simulink model "SecRwRtStFwdBkwdIsPosChk"  (R2024b)
settings: Solver=FixedStepDiscrete  StartTime=0.0  StopTime=10.0  FixedStep=0.01  RelTol=1e-3
undefined symbols (not defined in the file or in its folder): KeSMSuSecRwStFwdBkwdPosDelta_Val, KeSMSuSecRwStFwdBkwdPosTolr_Val
libraries: StIsPosChkLib x16, simulink x8
(part 1 of 2)
settings Model: Creator=sn2xws  LastModifiedBy=sn55gm
settings Model: ModifiedHistory=|
  | 2023.8.1 V2.0.0 CR421790 增加模式21-26
  | 2023.9.14 V2.1.0 Bug 540886 修改亲密模式判断到位的条件为10ms周期计算
  | 2023.11.16  V2.3.0 Issue 566045 全躺，vip，腿托打开增加前后位置
  | 2024.7.9 V3.0.0 557模式流程V1.9
  | 2024.8.15 V3.0.1 智享模式需要计算目标位置，不能直接判断到位置，posalready赋值0
  | 2024.9.5 V3.0.2 新增Md56，注释不用的模式
  | 2024.9.13 V3.0.3 6s版本lug不动二排前后
  | 2024.10.14 V3.0.4 新增Md57，md58
  | 2024.11.27 V3.0.5 Md57运行时，不能直接判断到位置
  | 25.7.1 V3.13.0 新增Md61 Md62
settings SolverCC: AlgebraicLoopSolver=TrustRegion
settings DataIOCC: SaveFormat=StructureWithTime  ReturnWorkspaceOutputs=off
settings OptimizationCC: DefaultParameterBehavior=Inlined  EnhancedBackFolding=on  PassReuseOutputArgsAs=Individual arguments  ZeroExternalMemoryAtStartup=off  ZeroInternalMemoryAtStartup=off  OptimizeBlockOrder=speed  DifferentSizesBufferReuse=on  OptimizationCustomize=off  EfficientTunableParamExpr=on
settings DebuggingCC: ParameterTunabilityLossMsg=error  UnconnectedInputMsg=warning  UnconnectedOutputMsg=warning  UnconnectedLineMsg=warning  ArithmeticOperatorsInVariantConditions=warning
settings ModelReferenceCC: EnableRefExpFcnMdlSchedulingChecks=on  ModelReferenceNumInstancesAllowed=Single
settings SFSimCC: MATLABDynamicMemAlloc=off  CustomCodeUndefinedFunction=UseInterfaceOnly
settings RTWCC: Description=AUTOSAR  SystemTargetFile=autosar.tlc  GenCodeOnly=on  TemplateMakefile=ert_default_tmf  GenerateReport=on  IncludeHyperlinkInReport=on  LaunchReport=on  DataTypeReplacement=CDataTypesFixedWidth  GenerateTraceInfo=on  GenerateTraceReport=on  GenerateTraceReportSl=on  GenerateTraceReportSf=on  GenerateTraceReportEml=on  GPUComputeCapability=3.5
settings CodeAppCC: ForceParamTrailComments=on  IgnoreCustomStorageClasses=off  OperatorAnnotations=on  SimulinkDataObjDesc=on  SFDataObjDesc=on  InsertBlockDesc=on
settings STFCustomTargetCC: TargetLangStandard=C99 (ISO)  MultiwordLength=256  ParMdlRefBuildCompliant=on  CompOptLevelCompliant=on  IncludeMdlTerminateFcn=off  CombineOutputUpdateFcns=on  SuppressErrorStatus=on  ERTCustomFileBanners=on  SupportNonFinite=off  SupportComplex=off  SupportContinuousTime=off  SupportNonInlinedSFcns=off  RemoveResetFunc=on  MATLABClassNameForMDSCustomization=Simulink.SoftwareTarget.ERTCustomization  AutosarCompliant=on  UseToolchainInfoCompliant=on  LookupTableObjectStructAxisOrder=2,1,3,4,...  LUTObjectStructOrderEvenSpacing=Size,Table,Breakpoints  SystemTargetFile=autosar.tlc
settings ERTTargetCC: TargetLangStandard=C99 (ISO)  ConcurrentExecutionCompliant=off  IncludeMdlTerminateFcn=off  SuppressErrorStatus=on  SupportNonFinite=off  SupportComplex=off  ModelStepFunctionPrototypeControlCompliant=off  CPPClassGenCompliant=off  AutosarCompliant=on  LookupTableObjectStructAxisOrder=2,1,3,4,...  LUTObjectStructOrderEvenSpacing=Size,Table,Breakpoints  ERTCustomFileTemplate=example_file_process.tlc  ERTFilePackagingFormat=Compact  BooleanTrueId=TRUE  BooleanFalseId=FALSE  DynamicArrayContainerType=coder::array

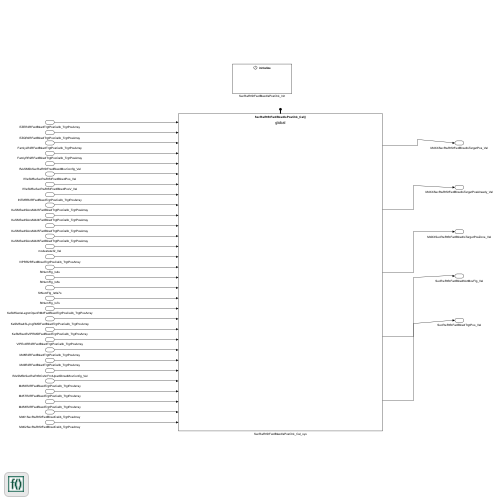
[thumbnail: Simulink's stored preview of the top-level diagram]
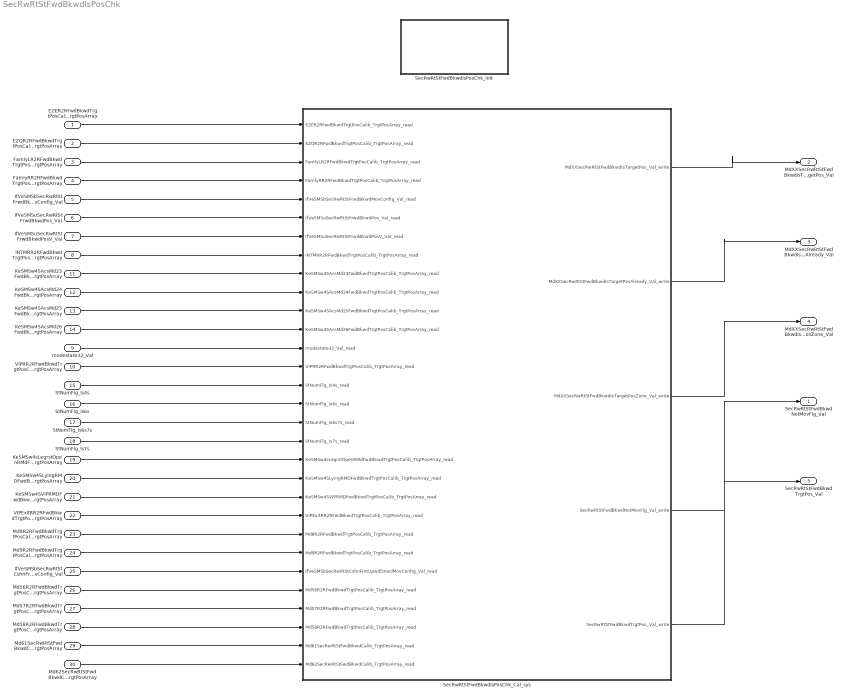
== system SecRwRtStFwdBkwdIsPosChk ==
  EZER2RFwdBkwdTrgtPosCalib_TrgtPosArray : Inport  Description=|  OutDataTypeStr=uint16  PortDimensions=3
      | 0:Pos
      | 1:Max
      | 2:Min
  EZQR2RFwdBkwdTrgtPosCalib_TrgtPosArray : Inport  Description=|  Port=2  OutDataTypeStr=uint16  PortDimensions=3
      | 0:Pos
      | 1:Max
      | 2:Min
  FamlyLR2RFwdBkwdTrgtPosCalib_TrgtPosArray : Inport  Description=|  Port=3  OutDataTypeStr=uint16  PortDimensions=3
      | 0:Pos
      | 1:Max
      | 2:Min
  FamlyRR2RFwdBkwdTrgtPosCalib_TrgtPosArray : Inport  Description=|  Port=4  OutDataTypeStr=uint16  PortDimensions=3
      | 0:Pos
      | 1:Max
      | 2:Min
  IfVeSMSbSecRwRtStFrwdBkwdMovConfig_Val : Inport  Port=5  OutDataTypeStr=boolean  PortDimensions=1
  IfVeSMSuSecRwRtStFrwdBkwdPos_Val : Inport  Port=6  OutDataTypeStr=uint16  PortDimensions=1
  IfVeSMSuSecRwRtStFrwdBkwdPosV_Val : Inport  Port=7  OutDataTypeStr=boolean  PortDimensions=1
  INTMRR2RFwdBkwdTrgtPosCalib_TrgtPosArray : Inport  Description=|  Port=8  OutDataTypeStr=uint16  PortDimensions=3
      | 0:Pos
      | 1:Max
      | 2:Min
  modestate32_Val : Inport  Port=9  OutDataTypeStr=uint32  PortDimensions=1
  VIPRR2RFwdBkwdTrgtPosCalib_TrgtPosArray : Inport  Description=|  Port=10  OutDataTypeStr=uint16  PortDimensions=3
      | 0:Pos
      | 1:Max
      | 2:Min
  KeSMSw4SAcsMd23FwdBkwdTrgtPosCalib_TrgtPosArray : Inport  Description=|  Port=11  OutDataTypeStr=uint16  PortDimensions=3
      | 0:Pos
      | 1:Max
      | 2:Min
  KeSMSw4SAcsMd24FwdBkwdTrgtPosCalib_TrgtPosArray : Inport  Description=|  Port=12  OutDataTypeStr=uint16  PortDimensions=3
      | 0:Pos
      | 1:Max
      | 2:Min
  KeSMSw4SAcsMd25FwdBkwdTrgtPosCalib_TrgtPosArray : Inport  Description=|  Port=13  OutDataTypeStr=uint16  PortDimensions=3
      | 0:Pos
      | 1:Max
      | 2:Min
  KeSMSw4SAcsMd26FwdBkwdTrgtPosCalib_TrgtPosArray : Inport  Description=|  Port=14  OutDataTypeStr=uint16  PortDimensions=3
      | 0:Pos
      | 1:Max
      | 2:Min
  StNumFlg_Is4s : Inport  Port=15  OutDataTypeStr=boolean  PortDimensions=1
  StNumFlg_Is6s : Inport  Port=16  OutDataTypeStr=boolean  PortDimensions=1
  StNumFlg_Is6s7s : Inport  Port=17  OutDataTypeStr=boolean  PortDimensions=1
  StNumFlg_Is7s : Inport  Port=18  OutDataTypeStr=boolean  PortDimensions=1
  KeSMSw4sLegrstOpenRMdFwdBkwdTrgtPosCalib_TrgtPosArray : Inport  Description=|  Port=19  OutDataTypeStr=uint16  PortDimensions=3
      | 0:Pos
      | 1:Max
      | 2:Min
  KeSMSw4SLyingRMDFwdBkwdTrgtPosCalib_TrgtPosArray : Inport  Description=|  Port=20  OutDataTypeStr=uint16  PortDimensions=3
      | 0:Pos
      | 1:Max
      | 2:Min
  KeSMSw4SVIPRMDFwdBkwdTrgtPosCalib_TrgtPosArray : Inport  Description=|  Port=21  OutDataTypeStr=uint16  PortDimensions=3
      | 0:Pos
      | 1:Max
      | 2:Min
  VIPExitRR2RFwdBkwdTrgtPosCalib_TrgtPosArray : Inport  Description=|  Port=22  OutDataTypeStr=uint16  PortDimensions=3
      | 0:Pos
      | 1:Max
      | 2:Min
  Md8R2RFwdBkwdTrgtPosCalib_TrgtPosArray : Inport  Description=|  Port=23  OutDataTypeStr=uint16  PortDimensions=3
      | 0:Pos
      | 1:Max
      | 2:Min
  Md9R2RFwdBkwdTrgtPosCalib_TrgtPosArray : Inport  Description=|  Port=24  OutDataTypeStr=uint16  PortDimensions=3
      | 0:Pos
      | 1:Max
      | 2:Min
  IfVeSMSbSecRwRtStCshnFrntUpwdDnwdMovConfig_Val : Inport  Port=25  OutDataTypeStr=boolean  PortDimensions=1
  Md56R2RFwdBkwdTrgtPosCalib_TrgtPosArray : Inport  Description=|  Port=26  OutDataTypeStr=uint16  PortDimensions=3
      | 0:Pos
      | 1:Max
      | 2:Min
  Md57R2RFwdBkwdTrgtPosCalib_TrgtPosArray : Inport  Description=|  Port=27  OutDataTypeStr=uint16  PortDimensions=3
      | 0:Pos
      | 1:Max
      | 2:Min
  Md58R2RFwdBkwdTrgtPosCalib_TrgtPosArray : Inport  Description=|  Port=28  OutDataTypeStr=uint16  PortDimensions=3
      | 0:Pos
      | 1:Max
      | 2:Min
  Md61SecRwRtStFwdBkwdCalib_TrgtPosArray : Inport  Description=|  Port=29  OutDataTypeStr=uint16  PortDimensions=3
      | 0:Pos
      | 1:Max
      | 2:Min
  Md62SecRwRtStFwdBkwdCalib_TrgtPosArray : Inport  Description=|  Port=30  OutDataTypeStr=uint16  PortDimensions=3
      | 0:Pos
      | 1:Max
      | 2:Min
  SecRwRtStFwdBkwdIsPosChk_Cal_sys : Subsystem
  SecRwRtStFwdBkwdIsPosChk_Init : Subsystem
  SecRwRtStFwdBkwdNotMovFlg_Val : Outport  OutDataTypeStr=boolean  PortDimensions=1  VectorParamsAs1DForOutWhenUnconnected=off
  MdXXSecRwRtStFwdBkwdIsTargetPos_Val : Outport  Port=2  OutDataTypeStr=uint32  PortDimensions=1  VectorParamsAs1DForOutWhenUnconnected=off
  MdXXSecRwRtStFwdBkwdIsTargetPosAlready_Val : Outport  Port=3  OutDataTypeStr=uint32  PortDimensions=1  VectorParamsAs1DForOutWhenUnconnected=off
  MdXXSecRwRtStFwdBkwdIsTargetPosZone_Val : Outport  Port=4  OutDataTypeStr=uint32  PortDimensions=1  VectorParamsAs1DForOutWhenUnconnected=off
  SecRwRtStFwdBkwdTrgtPos_Val : Outport  Port=5  OutDataTypeStr=uint16  PortDimensions=1  VectorParamsAs1DForOutWhenUnconnected=off
  wires:
  EZER2RFwdBkwdTrgtPosCalib_TrgtPosArray/1 -> SecRwRtStFwdBkwdIsPosChk_Cal_sys/1(EZER2RFwdBkwdTrgtPosCalib_TrgtPosArray_read)
  EZQR2RFwdBkwdTrgtPosCalib_TrgtPosArray/1 -> SecRwRtStFwdBkwdIsPosChk_Cal_sys/2(EZQR2RFwdBkwdTrgtPosCalib_TrgtPosArray_read)
  FamlyLR2RFwdBkwdTrgtPosCalib_TrgtPosArray/1 -> SecRwRtStFwdBkwdIsPosChk_Cal_sys/3(FamlyLR2RFwdBkwdTrgtPosCalib_TrgtPosArray_read)
  FamlyRR2RFwdBkwdTrgtPosCalib_TrgtPosArray/1 -> SecRwRtStFwdBkwdIsPosChk_Cal_sys/4(FamlyRR2RFwdBkwdTrgtPosCalib_TrgtPosArray_read)
  IfVeSMSbSecRwRtStFrwdBkwdMovConfig_Val/1 -> SecRwRtStFwdBkwdIsPosChk_Cal_sys/5(IfVeSMSbSecRwRtStFrwdBkwdMovConfig_Val_read)
  IfVeSMSuSecRwRtStFrwdBkwdPos_Val/1 -> SecRwRtStFwdBkwdIsPosChk_Cal_sys/6(IfVeSMSuSecRwRtStFrwdBkwdPos_Val_read)
  IfVeSMSuSecRwRtStFrwdBkwdPosV_Val/1 -> SecRwRtStFwdBkwdIsPosChk_Cal_sys/7(IfVeSMSuSecRwRtStFrwdBkwdPosV_Val_read)
  INTMRR2RFwdBkwdTrgtPosCalib_TrgtPosArray/1 -> SecRwRtStFwdBkwdIsPosChk_Cal_sys/8(INTMRR2RFwdBkwdTrgtPosCalib_TrgtPosArray_read)
  modestate32_Val/1 -> SecRwRtStFwdBkwdIsPosChk_Cal_sys/13(modestate32_Val_read)
  VIPRR2RFwdBkwdTrgtPosCalib_TrgtPosArray/1 -> SecRwRtStFwdBkwdIsPosChk_Cal_sys/14(VIPRR2RFwdBkwdTrgtPosCalib_TrgtPosArray_read)
  SecRwRtStFwdBkwdIsPosChk_Cal_sys/1(MdXXSecRwRtStFwdBkwdIsTargetPos_Val_write) -> MdXXSecRwRtStFwdBkwdIsTargetPos_Val/1
  SecRwRtStFwdBkwdIsPosChk_Cal_sys/2(MdXXSecRwRtStFwdBkwdIsTargetPosAlready_Val_write) -> MdXXSecRwRtStFwdBkwdIsTargetPosAlready_Val/1
  SecRwRtStFwdBkwdIsPosChk_Cal_sys/3(MdXXSecRwRtStFwdBkwdIsTargetPosZone_Val_write) -> MdXXSecRwRtStFwdBkwdIsTargetPosZone_Val/1
  SecRwRtStFwdBkwdIsPosChk_Cal_sys/4(SecRwRtStFwdBkwdNotMovFlg_Val_write) -> SecRwRtStFwdBkwdNotMovFlg_Val/1
  SecRwRtStFwdBkwdIsPosChk_Cal_sys/5(SecRwRtStFwdBkwdTrgtPos_Val_write) -> SecRwRtStFwdBkwdTrgtPos_Val/1
  KeSMSw4SAcsMd23FwdBkwdTrgtPosCalib_TrgtPosArray/1 -> SecRwRtStFwdBkwdIsPosChk_Cal_sys/9(KeSMSw4SAcsMd23FwdBkwdTrgtPosCalib_TrgtPosArray_read)
  KeSMSw4SAcsMd24FwdBkwdTrgtPosCalib_TrgtPosArray/1 -> SecRwRtStFwdBkwdIsPosChk_Cal_sys/10(KeSMSw4SAcsMd24FwdBkwdTrgtPosCalib_TrgtPosArray_read)
  KeSMSw4SAcsMd25FwdBkwdTrgtPosCalib_TrgtPosArray/1 -> SecRwRtStFwdBkwdIsPosChk_Cal_sys/11(KeSMSw4SAcsMd25FwdBkwdTrgtPosCalib_TrgtPosArray_read)
  KeSMSw4SAcsMd26FwdBkwdTrgtPosCalib_TrgtPosArray/1 -> SecRwRtStFwdBkwdIsPosChk_Cal_sys/12(KeSMSw4SAcsMd26FwdBkwdTrgtPosCalib_TrgtPosArray_read)
  StNumFlg_Is4s/1 -> SecRwRtStFwdBkwdIsPosChk_Cal_sys/15(StNumFlg_Is4s_read)
  StNumFlg_Is6s/1 -> SecRwRtStFwdBkwdIsPosChk_Cal_sys/16(StNumFlg_Is6s_read)
  StNumFlg_Is6s7s/1 -> SecRwRtStFwdBkwdIsPosChk_Cal_sys/17(StNumFlg_Is6s7s_read)
  StNumFlg_Is7s/1 -> SecRwRtStFwdBkwdIsPosChk_Cal_sys/18(StNumFlg_Is7s_read)
  KeSMSw4sLegrstOpenRMdFwdBkwdTrgtPosCalib_TrgtPosArray/1 -> SecRwRtStFwdBkwdIsPosChk_Cal_sys/19(KeSMSw4sLegrstOpenRMdFwdBkwdTrgtPosCalib_TrgtPosArray_read)
  KeSMSw4SLyingRMDFwdBkwdTrgtPosCalib_TrgtPosArray/1 -> SecRwRtStFwdBkwdIsPosChk_Cal_sys/20(KeSMSw4SLyingRMDFwdBkwdTrgtPosCalib_TrgtPosArray_read)
  KeSMSw4SVIPRMDFwdBkwdTrgtPosCalib_TrgtPosArray/1 -> SecRwRtStFwdBkwdIsPosChk_Cal_sys/21(KeSMSw4SVIPRMDFwdBkwdTrgtPosCalib_TrgtPosArray_read)
  VIPExitRR2RFwdBkwdTrgtPosCalib_TrgtPosArray/1 -> SecRwRtStFwdBkwdIsPosChk_Cal_sys/22(VIPExitRR2RFwdBkwdTrgtPosCalib_TrgtPosArray_read)
  Md8R2RFwdBkwdTrgtPosCalib_TrgtPosArray/1 -> SecRwRtStFwdBkwdIsPosChk_Cal_sys/23(Md8R2RFwdBkwdTrgtPosCalib_TrgtPosArray_read)
  Md9R2RFwdBkwdTrgtPosCalib_TrgtPosArray/1 -> SecRwRtStFwdBkwdIsPosChk_Cal_sys/24(Md9R2RFwdBkwdTrgtPosCalib_TrgtPosArray_read)
  IfVeSMSbSecRwRtStCshnFrntUpwdDnwdMovConfig_Val/1 -> SecRwRtStFwdBkwdIsPosChk_Cal_sys/25(IfVeSMSbSecRwRtStCshnFrntUpwdDnwdMovConfig_Val_read)
  Md56R2RFwdBkwdTrgtPosCalib_TrgtPosArray/1 -> SecRwRtStFwdBkwdIsPosChk_Cal_sys/26(Md56R2RFwdBkwdTrgtPosCalib_TrgtPosArray_read)
  Md57R2RFwdBkwdTrgtPosCalib_TrgtPosArray/1 -> SecRwRtStFwdBkwdIsPosChk_Cal_sys/27(Md57R2RFwdBkwdTrgtPosCalib_TrgtPosArray_read)
  Md58R2RFwdBkwdTrgtPosCalib_TrgtPosArray/1 -> SecRwRtStFwdBkwdIsPosChk_Cal_sys/28(Md58R2RFwdBkwdTrgtPosCalib_TrgtPosArray_read)
  Md61SecRwRtStFwdBkwdCalib_TrgtPosArray/1 -> SecRwRtStFwdBkwdIsPosChk_Cal_sys/29(Md61SecRwRtStFwdBkwdCalib_TrgtPosArray_read)
  Md62SecRwRtStFwdBkwdCalib_TrgtPosArray/1 -> SecRwRtStFwdBkwdIsPosChk_Cal_sys/30(Md62SecRwRtStFwdBkwdCalib_TrgtPosArray_read)

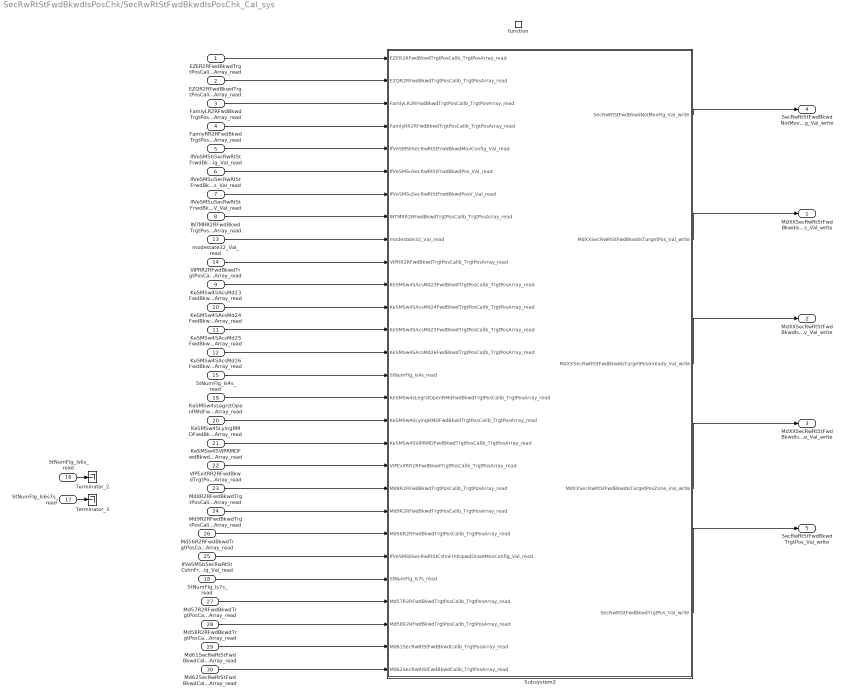
== system SecRwRtStFwdBkwdIsPosChk/SecRwRtStFwdBkwdIsPosChk_Cal_sys ==
  EZER2RFwdBkwdTrgtPosCalib_TrgtPosArray_read : Inport
  EZQR2RFwdBkwdTrgtPosCalib_TrgtPosArray_read : Inport  Port=2
  FamlyLR2RFwdBkwdTrgtPosCalib_TrgtPosArray_read : Inport  Port=3
  FamlyRR2RFwdBkwdTrgtPosCalib_TrgtPosArray_read : Inport  Port=4
  IfVeSMSbSecRwRtStFrwdBkwdMovConfig_Val_read : Inport  Port=5
  IfVeSMSuSecRwRtStFrwdBkwdPos_Val_read : Inport  Port=6
  IfVeSMSuSecRwRtStFrwdBkwdPosV_Val_read : Inport  Port=7
  INTMRR2RFwdBkwdTrgtPosCalib_TrgtPosArray_read : Inport  Port=8
  KeSMSw4SAcsMd23FwdBkwdTrgtPosCalib_TrgtPosArray_read : Inport  Port=9
  KeSMSw4SAcsMd24FwdBkwdTrgtPosCalib_TrgtPosArray_read : Inport  Port=10
  KeSMSw4SAcsMd25FwdBkwdTrgtPosCalib_TrgtPosArray_read : Inport  Port=11
  KeSMSw4SAcsMd26FwdBkwdTrgtPosCalib_TrgtPosArray_read : Inport  Port=12
  modestate32_Val_read : Inport  Port=13
  VIPRR2RFwdBkwdTrgtPosCalib_TrgtPosArray_read : Inport  Port=14
  StNumFlg_Is4s_read : Inport  Port=15
  StNumFlg_Is6s_read : Inport  Port=16
  StNumFlg_Is6s7s_read : Inport  Port=17
  StNumFlg_Is7s_read : Inport  Port=18
  KeSMSw4sLegrstOpenRMdFwdBkwdTrgtPosCalib_TrgtPosArray_read : Inport  Port=19
  KeSMSw4SLyingRMDFwdBkwdTrgtPosCalib_TrgtPosArray_read : Inport  Port=20
  KeSMSw4SVIPRMDFwdBkwdTrgtPosCalib_TrgtPosArray_read : Inport  Port=21
  VIPExitRR2RFwdBkwdTrgtPosCalib_TrgtPosArray_read : Inport  Port=22
  Md8R2RFwdBkwdTrgtPosCalib_TrgtPosArray_read : Inport  Port=23
  Md9R2RFwdBkwdTrgtPosCalib_TrgtPosArray_read : Inport  Port=24
  IfVeSMSbSecRwRtStCshnFrntUpwdDnwdMovConfig_Val_read : Inport  Port=25
  Md56R2RFwdBkwdTrgtPosCalib_TrgtPosArray_read : Inport  Port=26
  Md57R2RFwdBkwdTrgtPosCalib_TrgtPosArray_read : Inport  Port=27
  Md58R2RFwdBkwdTrgtPosCalib_TrgtPosArray_read : Inport  Port=28
  Md61SecRwRtStFwdBkwdCalib_TrgtPosArray_read : Inport  Port=29
  Md62SecRwRtStFwdBkwdCalib_TrgtPosArray_read : Inport  Port=30
  function : TriggerPort  TriggerType=function-call  IsSimulinkFunction=on  FunctionName=SecRwRtStFwdBkwdIsPosChk_Cal  VariantControl=(inherit)
  Subsystem2 : Subsystem
  Terminator_2 : Terminator
  Terminator_3 : Terminator
  MdXXSecRwRtStFwdBkwdIsTargetPos_Val_write : Outport  VectorParamsAs1DForOutWhenUnconnected=off
      settings: EnsureOutportIsVirtual=on
  MdXXSecRwRtStFwdBkwdIsTargetPosAlready_Val_write : Outport  Port=2  VectorParamsAs1DForOutWhenUnconnected=off
      settings: EnsureOutportIsVirtual=on
  MdXXSecRwRtStFwdBkwdIsTargetPosZone_Val_write : Outport  Port=3  VectorParamsAs1DForOutWhenUnconnected=off
      settings: EnsureOutportIsVirtual=on
  SecRwRtStFwdBkwdNotMovFlg_Val_write : Outport  Port=4  VectorParamsAs1DForOutWhenUnconnected=off
      settings: EnsureOutportIsVirtual=on
  SecRwRtStFwdBkwdTrgtPos_Val_write : Outport  Port=5  VectorParamsAs1DForOutWhenUnconnected=off
      settings: EnsureOutportIsVirtual=on
  wires:
  EZER2RFwdBkwdTrgtPosCalib_TrgtPosArray_read/1 -> Subsystem2/1(EZER2RFwdBkwdTrgtPosCalib_TrgtPosArray_read)
  EZQR2RFwdBkwdTrgtPosCalib_TrgtPosArray_read/1 -> Subsystem2/2(EZQR2RFwdBkwdTrgtPosCalib_TrgtPosArray_read)
  FamlyLR2RFwdBkwdTrgtPosCalib_TrgtPosArray_read/1 -> Subsystem2/3(FamlyLR2RFwdBkwdTrgtPosCalib_TrgtPosArray_read)
  FamlyRR2RFwdBkwdTrgtPosCalib_TrgtPosArray_read/1 -> Subsystem2/4(FamlyRR2RFwdBkwdTrgtPosCalib_TrgtPosArray_read)
  IfVeSMSbSecRwRtStFrwdBkwdMovConfig_Val_read/1 -> Subsystem2/5(IfVeSMSbSecRwRtStFrwdBkwdMovConfig_Val_read)
  IfVeSMSuSecRwRtStFrwdBkwdPos_Val_read/1 -> Subsystem2/6(IfVeSMSuSecRwRtStFrwdBkwdPos_Val_read)
  IfVeSMSuSecRwRtStFrwdBkwdPosV_Val_read/1 -> Subsystem2/7(IfVeSMSuSecRwRtStFrwdBkwdPosV_Val_read)
  INTMRR2RFwdBkwdTrgtPosCalib_TrgtPosArray_read/1 -> Subsystem2/8(INTMRR2RFwdBkwdTrgtPosCalib_TrgtPosArray_read)
  modestate32_Val_read/1 -> Subsystem2/9(modestate32_Val_read)
  VIPRR2RFwdBkwdTrgtPosCalib_TrgtPosArray_read/1 -> Subsystem2/10(VIPRR2RFwdBkwdTrgtPosCalib_TrgtPosArray_read)
  KeSMSw4SAcsMd23FwdBkwdTrgtPosCalib_TrgtPosArray_read/1 -> Subsystem2/11(KeSMSw4SAcsMd23FwdBkwdTrgtPosCalib_TrgtPosArray_read)
  KeSMSw4SAcsMd24FwdBkwdTrgtPosCalib_TrgtPosArray_read/1 -> Subsystem2/12(KeSMSw4SAcsMd24FwdBkwdTrgtPosCalib_TrgtPosArray_read)
  KeSMSw4SAcsMd25FwdBkwdTrgtPosCalib_TrgtPosArray_read/1 -> Subsystem2/13(KeSMSw4SAcsMd25FwdBkwdTrgtPosCalib_TrgtPosArray_read)
  KeSMSw4SAcsMd26FwdBkwdTrgtPosCalib_TrgtPosArray_read/1 -> Subsystem2/14(KeSMSw4SAcsMd26FwdBkwdTrgtPosCalib_TrgtPosArray_read)
  Subsystem2/1(SecRwRtStFwdBkwdNotMovFlg_Val_write) -> SecRwRtStFwdBkwdNotMovFlg_Val_write/1
  Subsystem2/5(SecRwRtStFwdBkwdTrgtPos_Val_write) -> SecRwRtStFwdBkwdTrgtPos_Val_write/1
  Subsystem2/2(MdXXSecRwRtStFwdBkwdIsTargetPos_Val_write) -> MdXXSecRwRtStFwdBkwdIsTargetPos_Val_write/1
  Subsystem2/4(MdXXSecRwRtStFwdBkwdIsTargetPosZone_Val_write) -> MdXXSecRwRtStFwdBkwdIsTargetPosZone_Val_write/1
  Subsystem2/3(MdXXSecRwRtStFwdBkwdIsTargetPosAlready_Val_write) -> MdXXSecRwRtStFwdBkwdIsTargetPosAlready_Val_write/1
  StNumFlg_Is4s_read/1 -> Subsystem2/15(StNumFlg_Is4s_read)
  StNumFlg_Is6s_read/1 -> Terminator_2/1
  StNumFlg_Is6s7s_read/1 -> Terminator_3/1
  StNumFlg_Is7s_read/1 -> Subsystem2/24(StNumFlg_Is7s_read)
  KeSMSw4sLegrstOpenRMdFwdBkwdTrgtPosCalib_TrgtPosArray_read/1 -> Subsystem2/16(KeSMSw4sLegrstOpenRMdFwdBkwdTrgtPosCalib_TrgtPosArray_read)
  KeSMSw4SLyingRMDFwdBkwdTrgtPosCalib_TrgtPosArray_read/1 -> Subsystem2/17(KeSMSw4SLyingRMDFwdBkwdTrgtPosCalib_TrgtPosArray_read)
  KeSMSw4SVIPRMDFwdBkwdTrgtPosCalib_TrgtPosArray_read/1 -> Subsystem2/18(KeSMSw4SVIPRMDFwdBkwdTrgtPosCalib_TrgtPosArray_read)
  VIPExitRR2RFwdBkwdTrgtPosCalib_TrgtPosArray_read/1 -> Subsystem2/19(VIPExitRR2RFwdBkwdTrgtPosCalib_TrgtPosArray_read)
  Md8R2RFwdBkwdTrgtPosCalib_TrgtPosArray_read/1 -> Subsystem2/20(Md8R2RFwdBkwdTrgtPosCalib_TrgtPosArray_read)
  Md9R2RFwdBkwdTrgtPosCalib_TrgtPosArray_read/1 -> Subsystem2/21(Md9R2RFwdBkwdTrgtPosCalib_TrgtPosArray_read)
  Md56R2RFwdBkwdTrgtPosCalib_TrgtPosArray_read/1 -> Subsystem2/22(Md56R2RFwdBkwdTrgtPosCalib_TrgtPosArray_read)
  IfVeSMSbSecRwRtStCshnFrntUpwdDnwdMovConfig_Val_read/1 -> Subsystem2/23(IfVeSMSbSecRwRtStCshnFrntUpwdDnwdMovConfig_Val_read)
  Md57R2RFwdBkwdTrgtPosCalib_TrgtPosArray_read/1 -> Subsystem2/25(Md57R2RFwdBkwdTrgtPosCalib_TrgtPosArray_read)
  Md58R2RFwdBkwdTrgtPosCalib_TrgtPosArray_read/1 -> Subsystem2/26(Md58R2RFwdBkwdTrgtPosCalib_TrgtPosArray_read)
  Md61SecRwRtStFwdBkwdCalib_TrgtPosArray_read/1 -> Subsystem2/27(Md61SecRwRtStFwdBkwdCalib_TrgtPosArray_read)
  Md62SecRwRtStFwdBkwdCalib_TrgtPosArray_read/1 -> Subsystem2/28(Md62SecRwRtStFwdBkwdCalib_TrgtPosArray_read)

== system SecRwRtStFwdBkwdIsPosChk/SecRwRtStFwdBkwdIsPosChk_Init ==
  note: Added blocks
  note: Added blocks
  Event Listener : EventListener  EventName=reset
  PA_KeSMSuSecRwStFwdBkwdPosDelta_Val : Constant  Value=KeSMSuSecRwStFwdBkwdPosDelta_Val
  PA_KeSMSuSecRwStFwdBkwdPosTolr_Val : Constant  Value=KeSMSuSecRwStFwdBkwdPosTolr_Val
  Terminator_1 : Terminator
  Terminator_2 : Terminator
  wires:
  PA_KeSMSuSecRwStFwdBkwdPosDelta_Val/1 -> Terminator_1/1
  PA_KeSMSuSecRwStFwdBkwdPosTolr_Val/1 -> Terminator_2/1

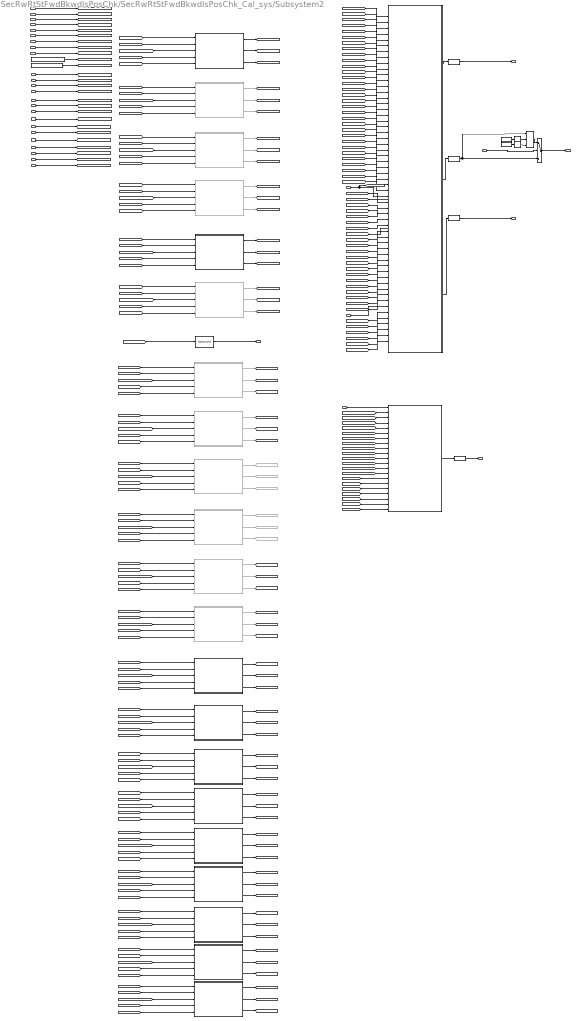
== system SecRwRtStFwdBkwdIsPosChk/SecRwRtStFwdBkwdIsPosChk_Cal_sys/Subsystem2 ==
  note: 2023.11.16 V2.3.0 Issue 566045 全躺，vip，腿托打开增加前后位置
  note: 2023.9.14 V2.1.0 Bug 540886 修改亲密模式判断到位的条件为10ms周期计算
  note: 2023.8.1 V2.0.0 CR421790 增加模式21-26
  EZER2RFwdBkwdTrgtPosCalib_TrgtPosArray_read : Inport
  EZQR2RFwdBkwdTrgtPosCalib_TrgtPosArray_read : Inport  Port=2
  FamlyLR2RFwdBkwdTrgtPosCalib_TrgtPosArray_read : Inport  Port=3
  FamlyRR2RFwdBkwdTrgtPosCalib_TrgtPosArray_read : Inport  Port=4
  IfVeSMSbSecRwRtStFrwdBkwdMovConfig_Val_read : Inport  Port=5
  IfVeSMSuSecRwRtStFrwdBkwdPos_Val_read : Inport  Port=6
  IfVeSMSuSecRwRtStFrwdBkwdPosV_Val_read : Inport  Port=7
  INTMRR2RFwdBkwdTrgtPosCalib_TrgtPosArray_read : Inport  Port=8
  modestate32_Val_read : Inport  Port=9
  VIPRR2RFwdBkwdTrgtPosCalib_TrgtPosArray_read : Inport  Port=10
  KeSMSw4SAcsMd23FwdBkwdTrgtPosCalib_TrgtPosArray_read : Inport  Port=11
  KeSMSw4SAcsMd24FwdBkwdTrgtPosCalib_TrgtPosArray_read : Inport  Port=12
  KeSMSw4SAcsMd25FwdBkwdTrgtPosCalib_TrgtPosArray_read : Inport  Port=13
  KeSMSw4SAcsMd26FwdBkwdTrgtPosCalib_TrgtPosArray_read : Inport  Port=14
  StNumFlg_Is4s_read : Inport  Port=15
  KeSMSw4sLegrstOpenRMdFwdBkwdTrgtPosCalib_TrgtPosArray_read : Inport  Port=16
  KeSMSw4SLyingRMDFwdBkwdTrgtPosCalib_TrgtPosArray_read : Inport  Port=17
  KeSMSw4SVIPRMDFwdBkwdTrgtPosCalib_TrgtPosArray_read : Inport  Port=18
  VIPExitRR2RFwdBkwdTrgtPosCalib_TrgtPosArray_read : Inport  Port=19
  Md8R2RFwdBkwdTrgtPosCalib_TrgtPosArray_read : Inport  Port=20
  Md9R2RFwdBkwdTrgtPosCalib_TrgtPosArray_read : Inport  Port=21
  Md56R2RFwdBkwdTrgtPosCalib_TrgtPosArray_read : Inport  Port=22
  IfVeSMSbSecRwRtStCshnFrntUpwdDnwdMovConfig_Val_read : Inport  Port=23
  StNumFlg_Is7s_read : Inport  Port=24
  Md57R2RFwdBkwdTrgtPosCalib_TrgtPosArray_read : Inport  Port=25
  Md58R2RFwdBkwdTrgtPosCalib_TrgtPosArray_read : Inport  Port=26
  Md61SecRwRtStFwdBkwdCalib_TrgtPosArray_read : Inport  Port=27
  Md62SecRwRtStFwdBkwdCalib_TrgtPosArray_read : Inport  Port=28
  Bitwise Operator : simulink/Logic and Bit Operations/Bitwise Operator  logicop=AND  UseBitMask=off  NumInputPorts=3  BitMask=bin2dec('11011001')  BitMaskRealWorld=Stored Integer
  Bitwise Operator1 : simulink/Logic and Bit Operations/Bitwise Operator  logicop=NOT  UseBitMask=off  BitMask=bin2dec('11011001')  BitMaskRealWorld=Stored Integer
  Bitwise Operator2 : simulink/Logic and Bit Operations/Bitwise Operator  logicop=NOT  UseBitMask=off  BitMask=bin2dec('11011001')  BitMaskRealWorld=Stored Integer
  Constant : Constant  Value=2048  OutDataTypeStr=uint32
  Constant1 : Constant  Value=1048576  OutDataTypeStr=uint32
  Data Type Conversion{,1..3} (4 alike) : DataTypeConversion  SaturateOnIntegerOverflow=off  RndMeth=Floor
  Goto40 : Goto  Commented=on  GotoTag=Md25IsTargetPosAlready
  Goto41 : Goto  Commented=on  GotoTag=Md25IsTargetPos
  Goto42 : Goto  Commented=on  GotoTag=Md25IsTargetPosZone
  Goto43 : Goto  Commented=on  GotoTag=Md26IsTargetPosAlready
  Goto44 : Goto  Commented=on  GotoTag=Md26IsTargetPos
  Goto45 : Goto  Commented=on  GotoTag=Md26IsTargetPosZone
  NotMovChk : StIsPosChkLib/NotMovChk  SystemSampleTime=-1  VariantActivationTime=update diagram  AllowFlexibleInterface=on  Latency=0  AutoFrameSizeCalculation=off
  PA_KeSMSuSecRwStFwdBkwdPosDelta_Val : Constant  Value=KeSMSuSecRwStFwdBkwdPosDelta_Val
  PA_KeSMSuSecRwStFwdBkwdPosTolr_Val : Constant  Value=KeSMSuSecRwStFwdBkwdPosTolr_Val
  Subsystem : Subsystem
  Subsystem1 : Subsystem
  Subsystem10 : Subsystem  Commented=on
  Subsystem11 : Subsystem  Commented=on
  Subsystem12 : Subsystem  Commented=on
  Subsystem13 : Subsystem  Commented=on
  Subsystem14 : Subsystem
  Subsystem15 : Subsystem
  Subsystem16 : Subsystem
  Subsystem17 : Subsystem
  Subsystem18 : Subsystem
  Subsystem19 : Subsystem
  Subsystem2 : Subsystem
  Subsystem20 : Subsystem
  Subsystem21 : Subsystem
  Subsystem22 : Subsystem
  Subsystem3 : Subsystem  Commented=on
  Subsystem4 : Subsystem  Commented=on
  Subsystem5 : Subsystem  Commented=on
  Subsystem6 : Subsystem
  Subsystem7 : Subsystem  Commented=on
  Subsystem8 : Subsystem  Commented=on
  Subsystem9 : Subsystem  Commented=on
  Switch : Switch  Criteria=u2 > Threshold  SaturateOnIntegerOverflow=off  InputSameDT=off
  SecRwRtStFwdBkwdNotMovFlg_Val_write : Outport  VectorParamsAs1DForOutWhenUnconnected=off
      settings: EnsureOutportIsVirtual=on
  MdXXSecRwRtStFwdBkwdIsTargetPos_Val_write : Outport  Port=2  VectorParamsAs1DForOutWhenUnconnected=off
      settings: EnsureOutportIsVirtual=on
  MdXXSecRwRtStFwdBkwdIsTargetPosAlready_Val_write : Outport  Port=3  VectorParamsAs1DForOutWhenUnconnected=off
      settings: EnsureOutportIsVirtual=on
  MdXXSecRwRtStFwdBkwdIsTargetPosZone_Val_write : Outport  Port=4  VectorParamsAs1DForOutWhenUnconnected=off
      settings: EnsureOutportIsVirtual=on
  SecRwRtStFwdBkwdTrgtPos_Val_write : Outport  Port=5  VectorParamsAs1DForOutWhenUnconnected=off
      settings: EnsureOutportIsVirtual=on
  wires:
  FamlyRR2RFwdBkwdTrgtPosCalib_TrgtPosArray_read/1 -> [FamlyRCalib]
  EZER2RFwdBkwdTrgtPosCalib_TrgtPosArray_read/1 -> [EZECalib]
  [PosDelta] -> Subsystem5/4(Delta)
  Subsystem7/3(IsPosAlready) -> [INTMLIsTargetPosAlready]
  Subsystem2/3(IsPosAlready) -> [EZEIsTargetPosAlready]
  [INTMLIsTargetPosZone] -> Subsystem1/19(INTMLIsTargetPosZone)
  Subsystem1/1(IsTargetPos) -> Data Type Conversion1/1
  [EZECalib] -> Subsystem2/3(CalibArray)
  [INTMLCalib] -> Subsystem7/3(CalibArray)
  INTMRR2RFwdBkwdTrgtPosCalib_TrgtPosArray_read/1 -> [INTMLCalib]
  [PosV] -> Subsystem6/1(PosV)
  Subsystem5/1(IsPos) -> [FamlyRIsTargetPos]
  Subsystem6/1(IsPos) -> [VIPLIsTargetPos]
  [PosTolr] -> Subsystem2/5(Tolr)
  [EZECalib] -> Subsystem/2(EZECalib)
  [Pos] -> NotMovChk/1
  Subsystem2/2(IsPosZone) -> [EZEIsTargetPosZone]
  [FamlyLCalib] -> Subsystem/4(FamlyLCalib)
  Subsystem3/2(IsPosZone) -> [EZQIsTargetPosZone]
  FamlyLR2RFwdBkwdTrgtPosCalib_TrgtPosArray_read/1 -> [FamlyLCalib]
  Subsystem4/3(IsPosAlready) -> [FamlyLIsTargetPosAlready]
  [FamlyLIsTargetPos] -> Subsystem1/4(FamlyLIsTargetPos)
  VIPRR2RFwdBkwdTrgtPosCalib_TrgtPosArray_read/1 -> [VIPLCalib]
  Subsystem7/1(IsPos) -> [INTMLIsTargetPos]
  [INTMLIsTargetPos] -> Subsystem1/7(INTMLIsTargetPos)
  [VIPLIsTargetPosAlready] -> Subsystem1/12(VIPLIsTargetPosAlready)
  [PosDelta] -> Subsystem4/4(Delta)
  [PosTolr] -> Subsystem7/5(Tolr)
  [VIPLCalib] -> Subsystem/6(VIPLCalib)
  Subsystem4/1(IsPos) -> [FamlyLIsTargetPos]
  [MovConfig] -> Subsystem1/1(MovConfig)
  Subsystem1/3(IsTargetPosZone) -> Data Type Conversion3/1
  [EZEIsTargetPosZone] -> Subsystem1/14(EZEIsTargetPosZone)
  [PosDelta] -> Subsystem7/4(Delta)
  PA_KeSMSuSecRwStFwdBkwdPosTolr_Val/1 -> [PosTolr]
  [Pos] -> Subsystem7/2(Pos)
  modestate32_Val_read/1 -> Subsystem/1(modestate32_Val_read)
  [PosDelta] -> Subsystem6/4(Delta)
  [EZQIsTargetPosZone] -> Subsystem1/15(EZQIsTargetPosZone)
  Subsystem6/2(IsPosZone) -> [VIPLIsTargetPosZone]
  Subsystem/1(TrgtPos) -> Data Type Conversion/1
  [FamlyLIsTargetPosZone] -> Subsystem1/16(FamlyLIsTargetPosZone)
  [INTMLIsTargetPosAlready] -> Subsystem1/13(INTMLIsTargetPosAlready)
  [VIPLCalib] -> Subsystem6/3(CalibArray)
  [VIPLIsTargetPosZone] -> Subsystem1/18(VIPLIsTargetPosZone)
  IfVeSMSbSecRwRtStFrwdBkwdMovConfig_Val_read/1 -> [MovConfig]
  [FamlyRIsTargetPosAlready] -> Subsystem1/11(FamlyRIsTargetPosAlready)
  [PosTolr] -> Subsystem5/5(Tolr)
  [FamlyLIsTargetPosAlready] -> Subsystem1/10(FamlyLIsTargetPosAlready)
  [FamlyRCalib] -> Subsystem/5(FamlyRCalib)
  [INTMLCalib] -> Subsystem/7(INTMLCalib)
  IfVeSMSuSecRwRtStFrwdBkwdPos_Val_read/1 -> [Pos]
  [FamlyRIsTargetPosZone] -> Subsystem1/17(FamlyRIsTargetPosZone)
  [PosV] -> Subsystem7/1(PosV)
  [FamlyRIsTargetPos] -> Subsystem1/5(FamlyRIsTargetPos)
  [FamlyLCalib] -> Subsystem4/3(CalibArray)
  [EZQCalib] -> Subsystem/3(EZQCalib)
  [EZQIsTargetPos] -> Subsystem1/3(EZQIsTargetPos)
  [EZEIsTargetPos] -> Subsystem1/2(EZEIsTargetPos)
  [EZEIsTargetPosAlready] -> Subsystem1/8(EZEIsTargetPosAlready)
  [Pos] -> Subsystem4/2(Pos)
  [Pos] -> Subsystem3/2(Pos)
  [EZQIsTargetPosAlready] -> Subsystem1/9(EZQIsTargetPosAlready)
  [EZQCalib] -> Subsystem3/3(CalibArray)
  PA_KeSMSuSecRwStFwdBkwdPosDelta_Val/1 -> [PosDelta]
  EZQR2RFwdBkwdTrgtPosCalib_TrgtPosArray_read/1 -> [EZQCalib]
  [PosTolr] -> Subsystem4/5(Tolr)
  [PosTolr] -> Subsystem6/5(Tolr)
  IfVeSMSuSecRwRtStFrwdBkwdPosV_Val_read/1 -> [PosV]
  Subsystem5/3(IsPosAlready) -> [FamlyRIsTargetPosAlready]
  [PosDelta] -> Subsystem2/4(Delta)
  Subsystem4/2(IsPosZone) -> [FamlyLIsTargetPosZone]
  [PosV] -> Subsystem5/1(PosV)
  Subsystem2/1(IsPos) -> [EZEIsTargetPos]
  [PosV] -> Subsystem2/1(PosV)
  [Pos] -> Subsystem5/2(Pos)
  NotMovChk/1 -> SecRwRtStFwdBkwdNotMovFlg_Val_write/1
  [PosV] -> Subsystem3/1(PosV)
  Subsystem3/3(IsPosAlready) -> [EZQIsTargetPosAlready]
  [PosDelta] -> Subsystem3/4(Delta)
  [PosTolr] -> Subsystem3/5(Tolr)
  [Pos] -> Subsystem2/2(Pos)
  [Pos] -> Subsystem6/2(Pos)
  [PosV] -> Subsystem4/1(PosV)
  Subsystem3/1(IsPos) -> [EZQIsTargetPos]
  Subsystem6/3(IsPosAlready) -> [VIPLIsTargetPosAlready]
  Subsystem1/2(IsTargetPosAlready) -> Data Type Conversion2/1
  Data Type Conversion1/1 -> MdXXSecRwRtStFwdBkwdIsTargetPos_Val_write/1
  Subsystem7/2(IsPosZone) -> [INTMLIsTargetPosZone]
  Data Type Conversion3/1 -> MdXXSecRwRtStFwdBkwdIsTargetPosZone_Val_write/1
  [VIPLIsTargetPos] -> Subsystem1/6(VIPLIsTargetPos)
  Subsystem5/2(IsPosZone) -> [FamlyRIsTargetPosZone]
  Data Type Conversion/1 -> SecRwRtStFwdBkwdTrgtPos_Val_write/1
  [FamlyRCalib] -> Subsystem5/3(CalibArray)
  KeSMSw4SAcsMd23FwdBkwdTrgtPosCalib_TrgtPosArray_read/1 -> [Md23Calib]
  KeSMSw4SAcsMd24FwdBkwdTrgtPosCalib_TrgtPosArray_read/1 -> [Md24Calib]
  KeSMSw4SAcsMd25FwdBkwdTrgtPosCalib_TrgtPosArray_read/1 -> [Md25Calib]
  KeSMSw4SAcsMd26FwdBkwdTrgtPosCalib_TrgtPosArray_read/1 -> [Md26Calib]
  Subsystem8/2(IsPosZone) -> [Md23IsTargetPosZone]
  [PosV] -> Subsystem8/1(PosV)
  [Pos] -> Subsystem8/2(Pos)
  [PosDelta] -> Subsystem8/4(Delta)
  [PosTolr] -> Subsystem8/5(Tolr)
  Subsystem8/1(IsPos) -> [Md23IsTargetPos]
  [Md23Calib] -> Subsystem8/3(CalibArray)
  Subsystem8/3(IsPosAlready) -> [Md23IsTargetPosAlready]
  Subsystem9/3(IsPosAlready) -> [Md24IsTargetPosAlready]
  [Md24Calib] -> Subsystem9/3(CalibArray)
  Subsystem9/1(IsPos) -> [Md24IsTargetPos]
  [PosTolr] -> Subsystem9/5(Tolr)
  [PosDelta] -> Subsystem9/4(Delta)
  [Pos] -> Subsystem9/2(Pos)
  [PosV] -> Subsystem9/1(PosV)
  Subsystem9/2(IsPosZone) -> [Md24IsTargetPosZone]
  Subsystem10/2(IsPosZone) -> Goto42/1
  [PosV] -> Subsystem10/1(PosV)
  [Pos] -> Subsystem10/2(Pos)
  [PosDelta] -> Subsystem10/4(Delta)
  [PosTolr] -> Subsystem10/5(Tolr)
  Subsystem10/1(IsPos) -> Goto41/1
  [Md25Calib] -> Subsystem10/3(CalibArray)
  Subsystem10/3(IsPosAlready) -> Goto40/1
  Subsystem11/3(IsPosAlready) -> Goto43/1
  [Md26Calib] -> Subsystem11/3(CalibArray)
  Subsystem11/1(IsPos) -> Goto44/1
  [PosTolr] -> Subsystem11/5(Tolr)
  [PosDelta] -> Subsystem11/4(Delta)
  [Pos] -> Subsystem11/2(Pos)
  [PosV] -> Subsystem11/1(PosV)
  Subsystem11/2(IsPosZone) -> Goto45/1
  [Md57Calib] -> Subsystem/8(Md57Calib)
  [Md58Calib] -> Subsystem/9(Md58Calib)
  [Md25Calib] -> Subsystem/10(Md25Calib)
  [Md26Calib] -> Subsystem/11(MD26Calib)
  [Md23IsTargetPos] -> Subsystem1/20(Md23IsTargetPos)
  [Md24IsTargetPos] -> Subsystem1/21(Md24IsTargetPos)
  [Md57IsTargetPos] -> Subsystem1/22(Md57IsTargetPos)
  [Md58IsTargetPos] -> Subsystem1/23(Md58IsTargetPos)
  [Md23IsTargetPosAlready] -> Subsystem1/24(Md23IsTargetPosAlready)
  [Md24IsTargetPosAlready] -> Subsystem1/25(Md24IsTargetPosAlready)
  [Md57IsTargetPosAlready] -> Subsystem1/26(Md57IsTargetPosAlready)
  [Md58IsTargetPosAlready] -> Subsystem1/27(Md58IsTargetPosAlready)
  [Md23IsTargetPosZone] -> Subsystem1/28(Md23IsTargetPosZone)
  [Md24IsTargetPosZone] -> Subsystem1/29(Md24IsTargetPosZone)
  [Md57IsTargetPosZone] -> Subsystem1/30(Md57IsTargetPosZone)
  [Md58IsTargetPosZone] -> Subsystem1/31(Md58IsTargetPosZone)
  StNumFlg_Is4s_read/1 -> [is4s], Subsystem1/32(StNumFlg_Is4s_read)
  KeSMSw4sLegrstOpenRMdFwdBkwdTrgtPosCalib_TrgtPosArray_read/1 -> [LgrstOpen4sCalib]
  KeSMSw4SLyingRMDFwdBkwdTrgtPosCalib_TrgtPosArray_read/1 -> [Ly4sCalib]
  KeSMSw4SVIPRMDFwdBkwdTrgtPosCalib_TrgtPosArray_read/1 -> [VIP4sCalib]
  Subsystem12/2(IsPosZone) -> [LgrstOpen4sIsTargetPosZone]
  [PosV] -> Subsystem12/1(PosV)
  [Pos] -> Subsystem12/2(Pos)
  [PosDelta] -> Subsystem12/4(Delta)
  [PosTolr] -> Subsystem12/5(Tolr)
  Subsystem12/1(IsPos) -> [LgrstOpen4sIsTargetPos]
  [LgrstOpen4sCalib] -> Subsystem12/3(CalibArray)
  Subsystem12/3(IsPosAlready) -> [LgrstOpen4sIsTargetPosAlready]
  Subsystem13/3(IsPosAlready) -> [Ly4sIsTargetPosAlready]
  [Ly4sCalib] -> Subsystem13/3(CalibArray)
  Subsystem13/1(IsPos) -> [Ly4sIsTargetPos]
  [PosTolr] -> Subsystem13/5(Tolr)
  [PosDelta] -> Subsystem13/4(Delta)
  [Pos] -> Subsystem13/2(Pos)
  [PosV] -> Subsystem13/1(PosV)
  Subsystem13/2(IsPosZone) -> [Ly4sIsTargetPosZone]
  Subsystem14/2(IsPosZone) -> [VIP4sIsTargetPosZone]
  [PosV] -> Subsystem14/1(PosV)
  [Pos] -> Subsystem14/2(Pos)
  [PosDelta] -> Subsystem14/4(Delta)
  [PosTolr] -> Subsystem14/5(Tolr)
  Subsystem14/1(IsPos) -> [VIP4sIsTargetPos]
  [VIP4sCalib] -> Subsystem14/3(CalibArray)
  Subsystem14/3(IsPosAlready) -> [VIP4sIsTargetPosAlready]
  [VIP4sCalib] -> Subsystem/12(VIP4sLCalib)
  [Ly4sCalib] -> Subsystem/13(Ly4sLCalib)
  [is4s] -> Subsystem/15(is4s)
  [LgrstOpen4sCalib] -> Subsystem/14(LgrstOpen4sLCalib)
  [VIP4sIsTargetPos] -> Subsystem1/33(VIP4sLIsTargetPos)
  [LgrstOpen4sIsTargetPos] -> Subsystem1/34(LgrstOpen4sLIsTargetPos)
  [Ly4sIsTargetPos] -> ?
  [VIP4sIsTargetPosAlready] -> Subsystem1/35(VIP4sLIsTargetPosAlready)
  [Ly4sIsTargetPosAlready] -> ?
  [LgrstOpen4sIsTargetPosAlready] -> Subsystem1/36(LgrstOpen4sLIsTargetPosAlready)
  [Ly4sIsTargetPosZone] -> ?
  [LgrstOpen4sIsTargetPosZone] -> Subsystem1/38(LgrstOpen4sLIsTargetPosZone)
  [VIP4sIsTargetPosZone] -> Subsystem1/37(VIP4sLIsTargetPosZone)
  VIPExitRR2RFwdBkwdTrgtPosCalib_TrgtPosArray_read/1 -> [Md28Calib]
  Subsystem15/3(IsPosAlready) -> [Md28IsTargetPosAlready]
  [Md28Calib] -> Subsystem15/3(CalibArray)
  Subsystem15/1(IsPos) -> [Md28IsTargetPos]
  [PosTolr] -> Subsystem15/5(Tolr)
  [PosDelta] -> Subsystem15/4(Delta)
  [Pos] -> Subsystem15/2(Pos)
  [PosV] -> Subsystem15/1(PosV)
  Subsystem15/2(IsPosZone) -> [Md28IsTargetPosZone]
  [Md28Calib] -> Subsystem/16(Md28Calib)
  [Md28IsTargetPos] -> Subsystem1/39(Md28IsTargetPos)
  [Md28IsTargetPosZone] -> Subsystem1/41(Md28IsTargetPosZone)
  [Md28IsTargetPosAlready] -> Subsystem1/40(Md28IsTargetPosAlready)
  Md8R2RFwdBkwdTrgtPosCalib_TrgtPosArray_read/1 -> [Md8Calib]
  Md9R2RFwdBkwdTrgtPosCalib_TrgtPosArray_read/1 -> [Md9Calib]
  Md56R2RFwdBkwdTrgtPosCalib_TrgtPosArray_read/1 -> [Md56Calib]
  Subsystem16/2(IsPosZone) -> [Md8IsTargetPosZone]
  [PosV] -> Subsystem16/1(PosV)
  [Pos] -> Subsystem16/2(Pos)
  [PosDelta] -> Subsystem16/4(Delta)
  [PosTolr] -> Subsystem16/5(Tolr)
  Subsystem16/1(IsPos) -> [Md8IsTargetPos]
  [Md8Calib] -> Subsystem16/3(CalibArray)
  Subsystem16/3(IsPosAlready) -> [Md8IsTargetPosAlready]
  Subsystem17/3(IsPosAlready) -> [Md9IsTargetPosAlready]
  [Md9Calib] -> Subsystem17/3(CalibArray)
  Subsystem17/1(IsPos) -> [Md9IsTargetPos]
  [PosTolr] -> Subsystem17/5(Tolr)
  [PosDelta] -> Subsystem17/4(Delta)
  [Pos] -> Subsystem17/2(Pos)
  [PosV] -> Subsystem17/1(PosV)
  Subsystem17/2(IsPosZone) -> [Md9IsTargetPosZone]
  Subsystem18/2(IsPosZone) -> [Md56IsTargetPosZone]
  [PosV] -> Subsystem18/1(PosV)
  [Pos] -> Subsystem18/2(Pos)
  [PosDelta] -> Subsystem18/4(Delta)
  [PosTolr] -> Subsystem18/5(Tolr)
  Subsystem18/1(IsPos) -> [Md56IsTargetPos]
  [Md56Calib] -> Subsystem18/3(CalibArray)
  Subsystem18/3(IsPosAlready) -> [Md56IsTargetPosAlready]
  [Md8Calib] -> Subsystem/17(Md8Calib)
  [Md9Calib] -> Subsystem/18(Md9Calib)
  [Md56Calib] -> Subsystem/19(Md56Calib)
  [Md8IsTargetPos] -> Subsystem1/42(Md8IsTargetPos)
  [Md9IsTargetPos] -> Subsystem1/43(Md9IsTargetPos)
  [Md56IsTargetPos] -> Subsystem1/44(Md56IsTargetPos)
  [Md8IsTargetPosAlready] -> Subsystem1/45(Md8IsTargetPosAlready)
  [Md9IsTargetPosAlready] -> Subsystem1/46(Md9IsTargetPosAlready)
  [Md56IsTargetPosAlready] -> Subsystem1/47(Md56IsTargetPosAlready)
  [Md8IsTargetPosZone] -> Subsystem1/48(Md8IsTargetPosZone)
  [Md9IsTargetPosZone] -> Subsystem1/49(Md9IsTargetPosZone)
  [Md56IsTargetPosZone] -> Subsystem1/50(Md56IsTargetPosZone)
  Constant/1 -> Bitwise Operator1/1
  Data Type Conversion2/1 -> Switch/3, Bitwise Operator/1
  IfVeSMSbSecRwRtStCshnFrntUpwdDnwdMovConfig_Val_read/1 -> Switch/2
  Switch/1 -> MdXXSecRwRtStFwdBkwdIsTargetPosAlready_Val_write/1
  Bitwise Operator1/1 -> Bitwise Operator/2
  Bitwise Operator/1 -> Switch/1
  StNumFlg_Is7s_read/1 -> Subsystem1/51(StNumFlg_Is7s_read)
  Md57R2RFwdBkwdTrgtPosCalib_TrgtPosArray_read/1 -> [Md57Calib]
  Md58R2RFwdBkwdTrgtPosCalib_TrgtPosArray_read/1 -> [Md58Calib]
  Subsystem19/3(IsPosAlready) -> [Md57IsTargetPosAlready]
  [Md57Calib] -> Subsystem19/3(CalibArray)
  Subsystem19/1(IsPos) -> [Md57IsTargetPos]
  [PosTolr] -> Subsystem19/5(Tolr)
  [PosDelta] -> Subsystem19/4(Delta)
  [Pos] -> Subsystem19/2(Pos)
  [PosV] -> Subsystem19/1(PosV)
  Subsystem19/2(IsPosZone) -> [Md57IsTargetPosZone]
  Subsystem20/2(IsPosZone) -> [Md58IsTargetPosZone]
  [PosV] -> Subsystem20/1(PosV)
  [Pos] -> Subsystem20/2(Pos)
  [PosDelta] -> Subsystem20/4(Delta)
  [PosTolr] -> Subsystem20/5(Tolr)
  Subsystem20/1(IsPos) -> [Md58IsTargetPos]
  [Md58Calib] -> Subsystem20/3(CalibArray)
  Subsystem20/3(IsPosAlready) -> [Md58IsTargetPosAlready]
  Constant1/1 -> Bitwise Operator2/1
  Bitwise Operator2/1 -> Bitwise Operator/3
  Md62SecRwRtStFwdBkwdCalib_TrgtPosArray_read/1 -> [Md62Calib]
  Md61SecRwRtStFwdBkwdCalib_TrgtPosArray_read/1 -> [Md61Calib]
  Subsystem21/3(IsPosAlready) -> [Md61IsTargetPosAlready]
  [Md61Calib] -> Subsystem21/3(CalibArray)
  Subsystem21/1(IsPos) -> [Md61IsTargetPos]
  [PosTolr] -> Subsystem21/5(Tolr)
  [PosDelta] -> Subsystem21/4(Delta)
  [Pos] -> Subsystem21/2(Pos)
  [PosV] -> Subsystem21/1(PosV)
  Subsystem21/2(IsPosZone) -> [Md61IsTargetPosZone]
  Subsystem22/2(IsPosZone) -> [Md62IsTargetPosZone]
  [PosV] -> Subsystem22/1(PosV)
  [Pos] -> Subsystem22/2(Pos)
  [PosDelta] -> Subsystem22/4(Delta)
  [PosTolr] -> Subsystem22/5(Tolr)
  Subsystem22/1(IsPos) -> [Md62IsTargetPos]
  [Md62Calib] -> Subsystem22/3(CalibArray)
  Subsystem22/3(IsPosAlready) -> [Md62IsTargetPosAlready]
  [Md62Calib] -> Subsystem/21(Md62Calib)
  [Md61Calib] -> Subsystem/20(Md61Calib)
  [Md61IsTargetPos] -> Subsystem1/52(Md61IsTargetPos)
  [Md62IsTargetPos] -> Subsystem1/53(Md62IsTargetPos)
  [Md61IsTargetPosAlready] -> Subsystem1/54(Md61IsTargetPosAlready)
  [Md62IsTargetPosAlready] -> Subsystem1/55(Md62IsTargetPosAlready)
  [Md61IsTargetPosZone] -> Subsystem1/56(Md61IsTargetPosZone)
  [Md62IsTargetPosZone] -> Subsystem1/57(Md62IsTargetPosZone)

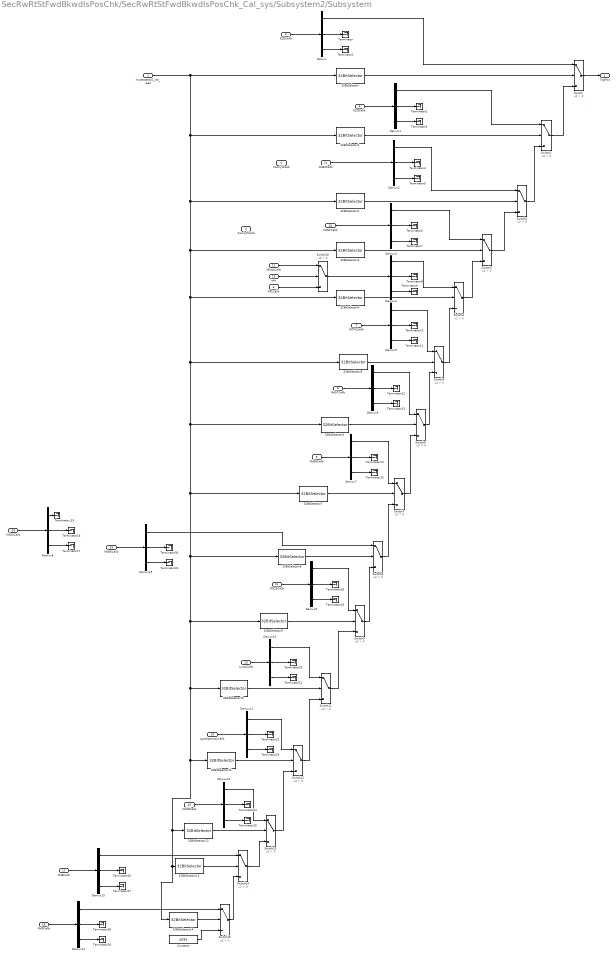
== system SecRwRtStFwdBkwdIsPosChk/SecRwRtStFwdBkwdIsPosChk_Cal_sys/Subsystem2/Subsystem ==
  modestate32_Val_read : Inport
  EZECalib : Inport  Port=2
  EZQCalib : Inport  Port=3
  FamlyLCalib : Inport  Port=4
  FamlyRCalib : Inport  Port=5
  VIPLCalib : Inport  Port=6
  INTMLCalib : Inport  Port=7
  Md57Calib : Inport  Port=8
  Md58Calib : Inport  Port=9
  Md25Calib : Inport  Port=10
  MD26Calib : Inport  Port=11
  VIP4sLCalib : Inport  Port=12
  Ly4sLCalib : Inport  Port=13
  LgrstOpen4sLCalib : Inport  Port=14
  is4s : Inport  Port=15
  Md28Calib : Inport  Port=16
  Md8Calib : Inport  Port=17
  Md9Calib : Inport  Port=18
  Md56Calib : Inport  Port=19
  Md61Calib : Inport  Port=20
  Md62Calib : Inport  Port=21
  32BitSelector : StIsPosChkLib/32BitSelector  BitNum=0
  32BitSelector1 : StIsPosChkLib/32BitSelector  BitNum=3
  32BitSelector10 : StIsPosChkLib/32BitSelector  BitNum=14
  32BitSelector11 : StIsPosChkLib/32BitSelector  BitNum=17
  32BitSelector12 : StIsPosChkLib/32BitSelector  BitNum=27
  32BitSelector13 : StIsPosChkLib/32BitSelector  BitNum=7
  32BitSelector14 : StIsPosChkLib/32BitSelector  BitNum=8
  32BitSelector2 : StIsPosChkLib/32BitSelector  BitNum=6
  32BitSelector3 : StIsPosChkLib/32BitSelector  BitNum=5
  32BitSelector4 : StIsPosChkLib/32BitSelector  BitNum=11
  32BitSelector5 : StIsPosChkLib/32BitSelector  BitNum=19
  32BitSelector6 : StIsPosChkLib/32BitSelector  BitNum=20
  32BitSelector7 : StIsPosChkLib/32BitSelector  BitNum=21
  32BitSelector8 : StIsPosChkLib/32BitSelector  BitNum=24
  32BitSelector9 : StIsPosChkLib/32BitSelector  BitNum=25
  Constant : Constant  Value=4095  OutDataTypeStr=uint16
  Demux{,1..15} (16 alike) : Demux  Outputs=3
  Switch{,1..15} (16 alike) : Switch  Criteria=u2 > Threshold  SaturateOnIntegerOverflow=off  InputSameDT=off
  Terminator{,1..31} (32 alike) : Terminator
  Terminator_33 : Terminator
  TrgtPos : Outport  VectorParamsAs1DForOutWhenUnconnected=off
      settings: EnsureOutportIsVirtual=on
  wires:
  32BitSelector/1 -> Switch/2
  Demux/1 -> Switch/1
  Demux/3 -> Terminator1/1
  Demux/2 -> Terminator/1
  EZECalib/1 -> Demux/1
  EZQCalib/1 -> Demux1/1
  Demux1/2 -> Terminator2/1
  Demux1/3 -> Terminator3/1
  Demux1/1 -> Switch1/1
  Switch/1 -> TrgtPos/1
  Switch1/1 -> Switch/3
  32BitSelector1/1 -> Switch1/2
  Switch2/1 -> Switch1/3
  Switch3/1 -> Switch2/3
  Switch4/1 -> Switch3/3
  32BitSelector2/1 -> Switch2/2
  32BitSelector3/1 -> Switch3/2
  32BitSelector4/1 -> Switch4/2
  Demux2/1 -> Switch2/1
  Demux2/3 -> Terminator5/1
  Demux2/2 -> Terminator4/1
  Demux3/2 -> Terminator6/1
  Demux3/3 -> Terminator7/1
  Demux3/1 -> Switch3/1
  Demux4/1 -> Switch4/1
  Demux4/3 -> Terminator9/1
  Demux4/2 -> Terminator8/1
  INTMLCalib/1 -> Demux5/1
  Demux5/2 -> Terminator10/1
  Demux5/3 -> Terminator11/1
  Demux5/1 -> Switch5/1
  Switch5/1 -> Switch4/3
  32BitSelector5/1 -> Switch5/2
  32BitSelector6/1 -> Switch6/2
  Switch6/1 -> Switch5/3
  Demux6/1 -> Switch6/1
  Demux6/3 -> Terminator13/1
  Demux6/2 -> Terminator12/1
  Md57Calib/1 -> Demux6/1
  Md58Calib/1 -> Demux7/1
  Demux7/2 -> Terminator14/1
  Demux7/3 -> Terminator15/1
  Demux7/1 -> Switch7/1
  Switch7/1 -> Switch6/3
  32BitSelector7/1 -> Switch7/2
  32BitSelector8/1 -> Switch8/2
  Switch8/1 -> Switch7/3
  Demux8/3 -> Terminator17/1
  Demux8/2 -> Terminator16/1
  Md25Calib/1 -> Demux8/1
  MD26Calib/1 -> Demux9/1
  Demux9/2 -> Terminator18/1
  Demux9/3 -> Terminator19/1
  Demux9/1 -> Switch9/1
  Switch9/1 -> Switch8/3
  32BitSelector9/1 -> Switch9/2
  is4s/1 -> Switch10/2
  VIP4sLCalib/1 -> Switch10/1
  VIPLCalib/1 -> Switch10/3
  Switch10/1 -> Demux4/1
  Switch11/1 -> Switch9/3
  Switch12/1 -> Switch11/3
  Demux10/1 -> Switch11/1
  Demux10/3 -> Terminator21/1
  Demux10/2 -> Terminator20/1
  Ly4sLCalib/1 -> Demux10/1
  LgrstOpen4sLCalib/1 -> Demux11/1
  Demux11/2 -> Terminator22/1
  Demux11/3 -> Terminator23/1
  Demux11/1 -> Switch12/1
  32BitSelector10/1 -> Switch11/2
  32BitSelector11/1 -> Switch12/2
  Switch13/1 -> Switch12/3
  32BitSelector12/1 -> Switch13/2
  Demux12/1 -> Switch13/1
  Demux12/3 -> Terminator25/1
  Demux12/2 -> Terminator24/1
  Md28Calib/1 -> Demux12/1
  modestate32_Val_read/1 -> 32BitSelector/1, 32BitSelector1/1, 32BitSelector2/1, 32BitSelector3/1, 32BitSelector4/1, 32BitSelector5/1, 32BitSelector6/1, 32BitSelector7/1, 32BitSelector8/1, 32BitSelector9/1, 32BitSelector14/1, 32BitSelector13/1, 32BitSelector12/1, 32BitSelector11/1, 32BitSelector10/1
  Switch14/1 -> Switch13/3
  Switch15/1 -> Switch14/3
  Constant/1 -> Switch15/3
  Demux13/1 -> Switch14/1
  Demux13/2 -> Terminator26/1
  Md8Calib/1 -> Demux13/1
  Demux13/3 -> Terminator27/1
  Demux14/3 -> Terminator29/1
  Md9Calib/1 -> Demux14/1
  Demux14/2 -> Terminator28/1
  Demux14/1 -> Switch15/1
  Demux15/2 -> Terminator30/1
  Md56Calib/1 -> Demux15/1
  Demux15/3 -> Terminator31/1
  32BitSelector13/1 -> Switch14/2
  32BitSelector14/1 -> Switch15/2
  Demux15/1 -> Switch8/1
  Demux8/1 -> Terminator_33/1
  Md61Calib/1 -> Demux3/1
  Md62Calib/1 -> Demux2/1
